simulink model "model2019a"  (R2019a)
settings: Solver=VariableStepAuto  StartTime=0.0  StopTime=50  RelTol=1e-3
libraries: fuzblock x3, dspnetwork x2, sldrtlib x1
settings Model: Creator=sopaj  LastModifiedBy=sopaj

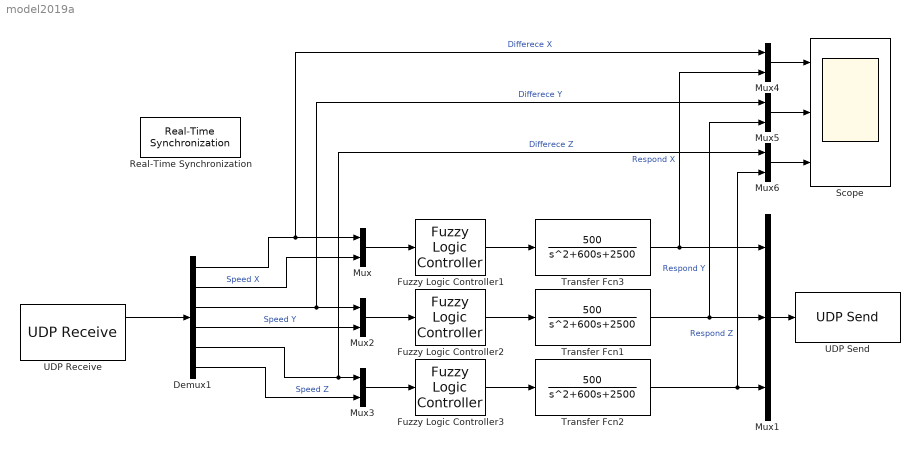
== system model2019a ==
  Demux1 : Demux  Outputs=6
  Fuzzy Logic Controller1 : fuzblock/Fuzzy Logic  Controller  FIS='final.fis'  OutputSampleNumber=101  DataType=double  FuzzifiedInputs=off  RuleFiringStrengths=off  RuleOutputs=off  AggregatedOutputs=off  SimulateUsing=Interpreted execution  OutOfRangeInputValueMessage=warning  NoRuleFiredMessage=warning  EmptyOutputFuzzySetMessage=warning
  Fuzzy Logic Controller2 : fuzblock/Fuzzy Logic  Controller  FIS='final.fis'  OutputSampleNumber=101  DataType=double  FuzzifiedInputs=off  RuleFiringStrengths=off  RuleOutputs=off  AggregatedOutputs=off  SimulateUsing=Interpreted execution  OutOfRangeInputValueMessage=warning  NoRuleFiredMessage=warning  EmptyOutputFuzzySetMessage=warning
  Fuzzy Logic Controller3 : fuzblock/Fuzzy Logic  Controller  FIS='final.fis'  OutputSampleNumber=101  DataType=double  FuzzifiedInputs=off  RuleFiringStrengths=off  RuleOutputs=off  AggregatedOutputs=off  SimulateUsing=Interpreted execution  OutOfRangeInputValueMessage=warning  NoRuleFiredMessage=warning  EmptyOutputFuzzySetMessage=warning
  Mux{,2..6} (6 alike) : Mux  Inputs=2
  Mux1 : Mux  Inputs=3
  Real-Time Synchronization : sldrtlib/Real-Time Synchronization  SampleTime=0.01  MaxMissedTicks=100  ShowMissedTicks=off  YieldWhenWaiting=off
  Scope : Scope  NumInputPorts=3
  Transfer Fcn1 : TransferFcn  Numerator=[500]  Denominator=[1 600 2500]
  Transfer Fcn2 : TransferFcn  Numerator=[500]  Denominator=[1 600 2500]
  Transfer Fcn3 : TransferFcn  Numerator=[500]  Denominator=[1 600 2500]
  UDP Receive : dspnetwork/UDP Receive  localURL='0.0.0.0'  localPort=25001  remoteURL='0.0.0.0'  remotePort=-1  recvBufferSize=8192  dims=6  signalDatatype=double  isComplex=off  isVarSize=off  showBlockingTime=off  blockingTime=0  sampletime=0.01  blockPlatform=[]
  UDP Send : dspnetwork/UDP Send  remoteURL='127.0.0.1'  remotePort=25000  localURL='0.0.0.0'  localPortSource=Automatically determine  localPort=-1  sampletime=-1  blockPlatform=[]  separateLengthPort=0
  wires:
  UDP Receive/1 -> Demux1/1
  Mux1/1 -> UDP Send/1
  Fuzzy Logic Controller1/1 -> Transfer Fcn3/1
  Mux/1 -> Fuzzy Logic Controller1/1
  Mux2/1 -> Fuzzy Logic Controller2/1
  Mux3/1 -> Fuzzy Logic Controller3/1
  Fuzzy Logic Controller2/1 -> Transfer Fcn1/1
  Fuzzy Logic Controller3/1 -> Transfer Fcn2/1
  Mux6/1 -> Scope/3
  Mux5/1 -> Scope/2
  Mux4/1 -> Scope/1
  Demux1/3 -> Mux5/1, Mux2/1  "Differece Y"
  Demux1/4 -> Mux2/2  "Speed Y"
  Demux1/2 -> Mux/2  "Speed X"
  Demux1/1 -> Mux4/1, Mux/1  "Differece X"
  Demux1/5 -> Mux6/1, Mux3/1  "Differece Z"
  Demux1/6 -> Mux3/2  "Speed Z"
  Transfer Fcn2/1 -> Mux6/2, Mux1/3  "Respond Z"
  Transfer Fcn1/1 -> Mux5/2, Mux1/2  "Respond Y"
  Transfer Fcn3/1 -> Mux4/2, Mux1/1  "Respond X"
